simulink model "feedback_control"  (R2020b)
settings: Solver=FixedStepDiscrete  StartTime=0.0  StopTime=inf  FixedStep=T_sample_control  RelTol=1e-3  EnableMultiTasking=on
undefined symbols (not defined in the file): T_sample_control
libraries: dspstat3 x1
settings Model: DataDictionary=pid.sldd  EnableAccessToBaseWorkspace=off  ModifiedByFormat=The MathWorks Inc.  Creator=The MathWorks, Inc.  LastModifiedBy=The MathWorks Inc.
settings DataIOCC: SaveFormat=Array  ReturnWorkspaceOutputs=off
settings OptimizationCC: DefaultParameterBehavior=Inlined  InlineInvariantSignals=on  PassReuseOutputArgsAs=Individual arguments  ExpressionDepthLimit=2147483647  EfficientFloat2IntCast=on  LifeSpan=1  EfficientTunableParamExpr=on
settings DebuggingCC: SolverPrmCheckMsg=warning  FcnCallInpInsideContextMsg=warning  UniqueDataStoreMsg=error  AssertControl=DisableAll  AllowSymbolicDim=off  StateNameClashWarn=warning  StrictBusMsg=ErrorOnBusTreatedAsVector  SFUnexpectedBacktrackingDiag=warning  SFNoUnconditionalDefaultTransitionDiag=warning  SFExecutionAtInitializationDiag=none  ArithmeticOperatorsInVariantConditions=warning
settings HardwareCC: ProdBitPerPointer=32  ProdBitPerSizeT=32  ProdBitPerPtrDiffT=32  ProdLargestAtomicInteger=Long  ProdLargestAtomicFloat=Double  ProdWordSize=32  ProdHWDeviceType=ARM Compatible->ARM Cortex-M
settings ModelReferenceCC: PropagateSignalLabelsOutOfModel=off
settings SFSimCC: SimUseLocalCustomCode=off  CustomCodeUndefinedFunction=UseInterfaceOnly
settings RTWCC: Description=Embedded Coder  SystemTargetFile=ert.tlc  GenCodeOnly=on  TemplateMakefile=ert_default_tmf  GenerateReport=on  RTWUseLocalCustomCode=off  IncludeHyperlinkInReport=on  LaunchReport=on  GenerateTraceInfo=on  GenerateTraceReport=on  GenerateTraceReportSl=on  GenerateTraceReportSf=on  GenerateTraceReportEml=on  GenerateCodeMetricsReport=on
settings CodeAppCC: IgnoreCustomStorageClasses=off  IgnoreTestpoints=on  CustomSymbolStrType=$N$R$M  StateflowObjectComments=on  InternalIdentifier=Classic
settings ERTTargetCC: MultiwordLength=2048  GenerateSampleERTMain=on  CodeInterfacePackaging=Reusable function  SupportNonFinite=off  ParenthesesLevel=Maximum  InlinedParameterPlacement=NonHierarchical  ERTCustomFileTemplate=example_file_process.tlc  ERTFilePackagingFormat=Compact  ConvertIfToSwitch=off  SuppressUnreachableDefaultCases=off
settings ConfigComp: CovMetricSettings=dw  CovSaveCumulativeToWorkspaceVar=on  CovSaveSingleToWorkspaceVar=on  CovExternalEMLEnable=off  CovSFcnEnable=off

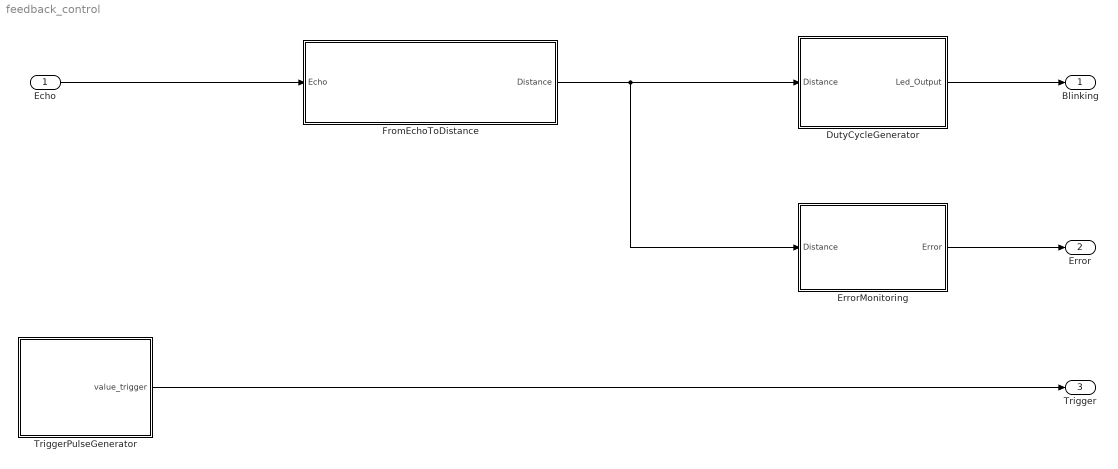
== system feedback_control ==
  Echo : Inport  PortDimensions=1  SampleTime=T_sample_control
  DutyCycleGenerator : Subsystem
  ErrorMonitoring : Subsystem
  FromEchoToDistance : Subsystem
  TriggerPulseGenerator : Subsystem
  Blinking : Outport  OutDataTypeStr=boolean  PortDimensions=1  SampleTime=T_sample_control
  Error : Outport  Port=2  OutDataTypeStr=boolean
  Trigger : Outport  Port=3  OutDataTypeStr=boolean
  wires:
  DutyCycleGenerator/1(Led_Output) -> Blinking/1
  ErrorMonitoring/1(Error) -> Error/1
  FromEchoToDistance/1(Distance) -> ErrorMonitoring/1(Distance), DutyCycleGenerator/1(Distance)
  Echo/1 -> FromEchoToDistance/1(Echo)
  TriggerPulseGenerator/1(value_trigger) -> Trigger/1

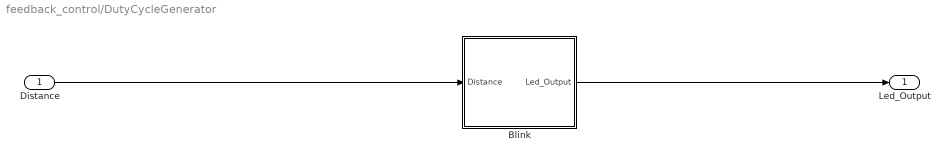
== system feedback_control/DutyCycleGenerator ==
  Distance : Inport  OutDataTypeStr=double
  Blink : Stateflow chart  TreatAsAtomicUnit=on
  Led_Output : Outport  OutDataTypeStr=boolean
  wires:
  Distance/1 -> Blink/1(Distance)
  Blink/1(Led_Output) -> Led_Output/1

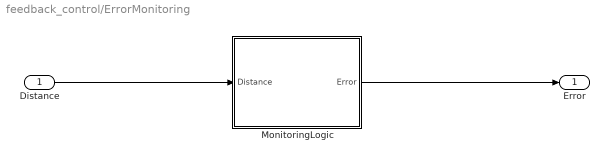
== system feedback_control/ErrorMonitoring ==
  Distance : Inport  OutDataTypeStr=double
  MonitoringLogic : Stateflow chart  TreatAsAtomicUnit=on
  Error : Outport  OutDataTypeStr=boolean
  wires:
  Distance/1 -> MonitoringLogic/1(Distance)
  MonitoringLogic/1(Error) -> Error/1

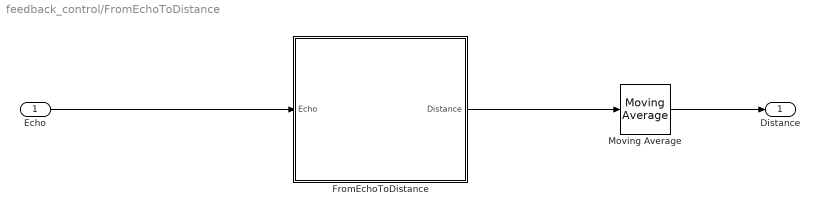
== system feedback_control/FromEchoToDistance ==
  Echo : Inport
  FromEchoToDistance : Stateflow chart  TreatAsAtomicUnit=on
  Moving Average : dspstat3/Moving Average  Method=Sliding window  ForgettingFactorPort=off  SpecifyWindowLength=on  WindowLength=4  ForgettingFactor=0.9  SimulateUsing=Code generation
  Distance : Outport
  wires:
  Echo/1 -> FromEchoToDistance/1(Echo)
  Moving Average/1 -> Distance/1
  FromEchoToDistance/1(Distance) -> Moving Average/1

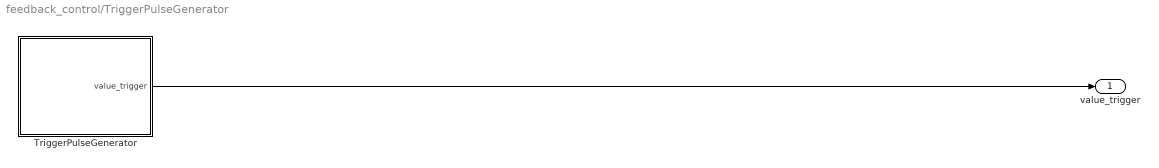
== system feedback_control/TriggerPulseGenerator ==
  TriggerPulseGenerator : Stateflow chart  TreatAsAtomicUnit=on
  value_trigger : Outport
  wires:
  TriggerPulseGenerator/1(value_trigger) -> value_trigger/1

== stateflow chart feedback_control/ErrorMonitoring/MonitoringLogic ==
  state RESET
    en: Error=false;
  note: stato iniziale assumiamo nessun errore
  state CHECK_FOR_ERROR
    en: Error=false;
  state ERROR_STATE
    en: Error=true;
  (default) -> RESET
  (junction 13) -> RESET
  (junction 11) -> (junction 13)
  RESET -> CHECK_FOR_ERROR : [((Distance<2) || (Distance >400)) && Distance~=0]
  CHECK_FOR_ERROR -> (junction 11) [order 1] : [(Distance>=2) && (Distance <=400)]
  (junction 23) -> (junction 11)
  CHECK_FOR_ERROR -> ERROR_STATE [order 2] : after(400,msec)[((Distance<2) || (Distance>400) && Distance ~=0)]
  ERROR_STATE -> (junction 23) : [(Distance>=2) && (Distance <=400) || Distance==0]
  data: Distance input double; Error output boolean

== stateflow chart feedback_control/TriggerPulseGenerator/TriggerPulseGenerator ==
  state HIGH
    en: value_trigger =true;
  note: Trigger pulse every 100ms
  state LOW
    en: value_trigger =false;
  (default) -> HIGH
  LOW -> HIGH : after(100000-2,usec)
  HIGH -> LOW : after(20,usec)
  data: value_trigger output boolean

== stateflow chart feedback_control/FromEchoToDistance/FromEchoToDistance ==
  state COMPUTE_ECHO_DURATION [parallel]
    settings: executionOrder=1
    state INIT
      en: Counter=0;
    state WAIT_TO_FALL
      en: Counter = Counter + 1;
    (default) -> INIT
    INIT -> INIT [order 2] : after(100,msec)[Echo==0]{Distance=0;}
    WAIT_TO_FALL -> INIT [order 2] : {Distance=Counter/58;}
    INIT -> WAIT_TO_FALL [order 1] : [Echo==1]
    WAIT_TO_FALL -> WAIT_TO_FALL [order 1] : [Echo==1]
  data: Echo input double; Distance output double; Counter local double

== stateflow chart feedback_control/DutyCycleGenerator/Blink ==
  state NO_BLINK
  state Blinker2
    state LED_ON
      en: Led_Output=true;
    state LED_OFF
      en: Led_Output=false;
    (default) -> Blinker2.LED_ON
    Blinker2.LED_OFF -> Blinker2.LED_ON : after(250,msec)
    Blinker2.LED_ON -> Blinker2.LED_OFF : after(250,msec)
  state blinker3
    state LED_ON
      en: Led_Output=true;
    state LED_OFF
      en: Led_Output=false;
    (default) -> blinker3.LED_ON
    blinker3.LED_OFF -> blinker3.LED_ON : after(500,msec)
    blinker3.LED_ON -> blinker3.LED_OFF : after(500,msec)
  state Blinker1
    state LED_ON
      en: Led_Output=true;
    state LED_OFF
      en: Led_Output=false;
    Blinker1.LED_ON -> Blinker1.LED_ON [order 1] : [Distance==100]
    (default) -> Blinker1.LED_ON
    Blinker1.LED_OFF -> Blinker1.LED_ON : after(0.1-Distance/1000, sec)
    Blinker1.LED_ON -> Blinker1.LED_OFF [order 2] : after(Distance/1000, sec)
  (default) -> NO_BLINK
  NO_BLINK -> (junction 17) [order 1] : [Distance>=10 && Distance <=100]
  (junction 46) -> NO_BLINK
  blinker3 -> (junction 46) : [Distance~=0]
  (junction 17) -> Blinker1
  NO_BLINK -> (junction 41) [order 3]
  (junction 41) -> blinker3
  (junction 23) -> NO_BLINK
  Blinker1 -> (junction 23) : [Distance<10 || Distance >100]
  NO_BLINK -> Blinker2 [order 2] : [((Distance<10 )|| (Distance>100)) && Distance~=0]
  Blinker2 -> NO_BLINK : [(Distance>=10 && Distance<=100) || Distance==0]
  data: Distance input double; Led_Output output boolean
